simulink subsystem "TX"  (R2022b)
settings: Solver=VariableStepAuto  StartTime=0.0  StopTime=10.0  RelTol=1e-3
settings Model: Creator=Ali-Laptop  LastModifiedBy=Ali-Laptop

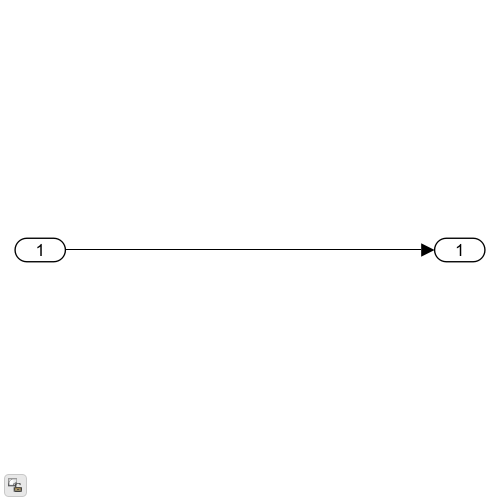
[thumbnail: Simulink's stored preview of the top-level diagram]
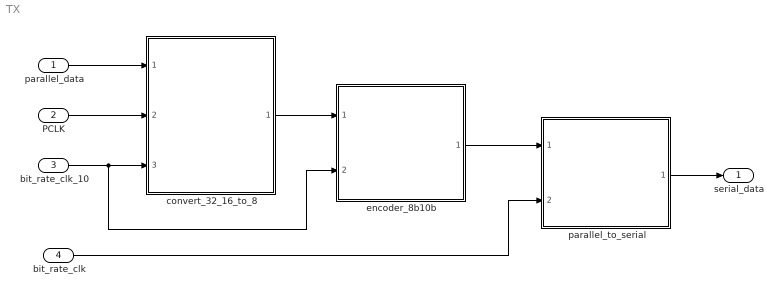
== system TX ==
  parallel_data : Inport
  PCLK : Inport  Port=2
  bit_rate_clk_10 : Inport  Port=3
  bit_rate_clk : Inport  Port=4
  convert_32_16_to_8 : Subsystem  ReferencedSubsystem=convert_32_16_to_8
  encoder_8b10b : Subsystem  ReferencedSubsystem=encoder_8b10b
  parallel_to_serial : Subsystem  ReferencedSubsystem=parallel_to_serial
  serial_data : Outport
  wires:
  parallel_to_serial/1 -> serial_data/1
  parallel_data/1 -> convert_32_16_to_8/1
  PCLK/1 -> convert_32_16_to_8/2
  convert_32_16_to_8/1 -> encoder_8b10b/1
  bit_rate_clk_10/1 -> encoder_8b10b/2, convert_32_16_to_8/3
  bit_rate_clk/1 -> parallel_to_serial/2
  encoder_8b10b/1 -> parallel_to_serial/1
